simulink library "ForcesSubsystem"  (R2021b)
settings: Solver=VariableStepAuto  StartTime=0.0  StopTime=10.0  RelTol=1e-3
undefined symbols (not defined in the file): sigbuilder_block
libraries: gravitySubsystem x1
settings Model: Creator=mat  LastModifiedBy=mat

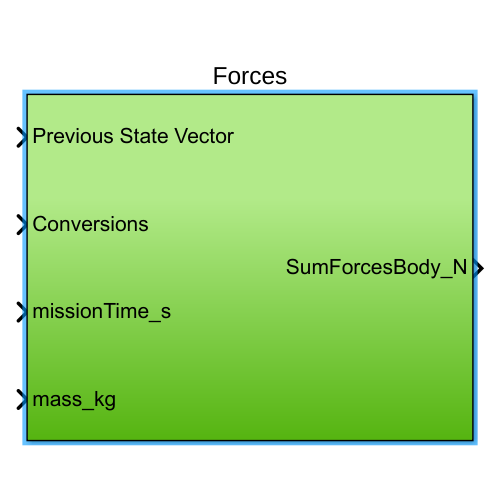
[thumbnail: Simulink's stored preview of the top-level diagram]
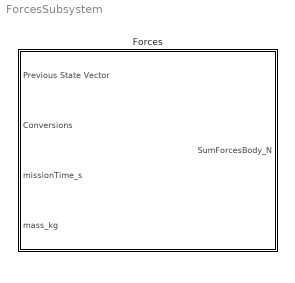
== system ForcesSubsystem ==
  Forces : Subsystem

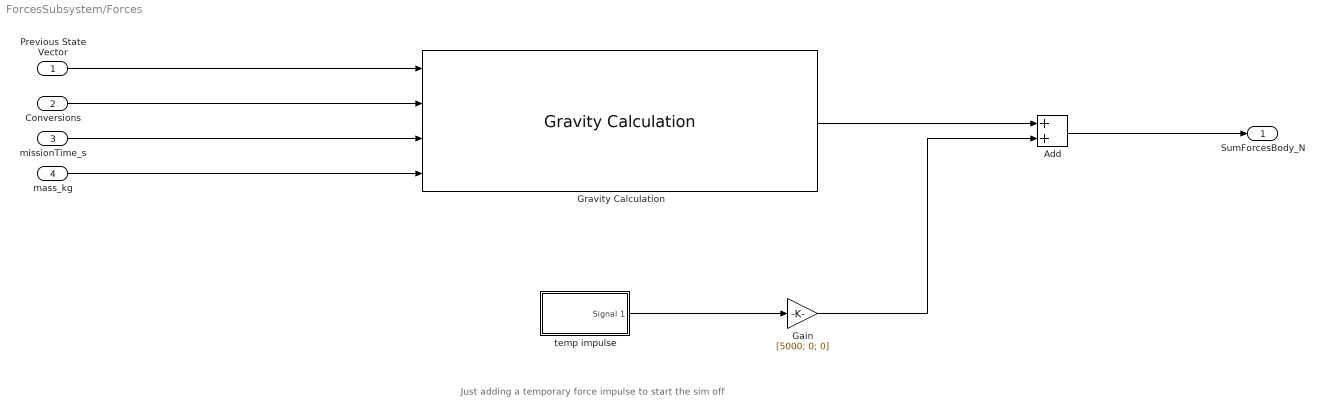
== system ForcesSubsystem/Forces ==
  note: Just adding a temporary force impulse to start the sim off
  Previous State Vector : Inport  OutDataTypeStr=Bus: StateVector_BusType
  Conversions : Inport  Port=2  OutDataTypeStr=Bus: Conversions_BusType
  missionTime_s : Inport  Port=3
  mass_kg : Inport  Port=4
  Add : Sum  InputSameDT=on
  Gain : Gain  Gain=[5000; 0; 0]
  Gravity Calculation : gravitySubsystem/Gravity Calculation  SystemSampleTime=-1  VariantActivationTime=update diagram  Latency=0  AutoFrameSizeCalculation=off
  temp impulse : Subsystem  Tag=STV Subsys  LoadFcn=sigbuilder_block('load');  StartFcn=sigbuilder_block('start');  StopFcn=sigbuilder_block('stop');  ClipboardFcn=sigbuilder_block('clipboard');  mask(Sigbuilder block){tuvar=[0:10]}
      mask help: Simulink:masks:SigbuilderBlock_MD
      mask init:
      | if ~strcmp(get_param(bdroot(gcbh),'SimulationStatus'),'stopped') tuvar = sigbuilder_block('maskInit'); end
      settings: CopyFcn=sigbuilder_block('copy');  DeleteFcn=sigbuilder_block('delete');  ModelCloseFcn=sigbuilder_block('modelClose');  PreSaveFcn=sigbuilder_block('preSave');  PauseFcn=sigbuilder_block('pause');  ContinueFcn=sigbuilder_block('continue');  NameChangeFcn=sigbuilder_block('namechange');  OpenFcn=sigbuilder_block('open',[0 0 1561.26 692.716 ]);  CloseFcn=sigbuilder_block('close');
      mask Display: plot(0, 0, 100, 100,[2, 2, 32, 32, 2], [68, 8, 8, 68, 68],[32, 2], [38, 38], [32, 19, 2],[53, 60, 44], [32, 17, 17, 2],[16, 16, 31, 31]);txt = getActiveGroup(gcbh);text(2, 100, txt,'verticalAlignment', 'top');
  SumForcesBody_N : Outport
  wires:
  mass_kg/1 -> Gravity Calculation/4
  missionTime_s/1 -> Gravity Calculation/3
  Gravity Calculation/1 -> Add/1
  Conversions/1 -> Gravity Calculation/2
  Previous State Vector/1 -> Gravity Calculation/1
  temp impulse/1(Signal 1) -> Gain/1
  Gain/1 -> Add/2
  Add/1 -> SumForcesBody_N/1

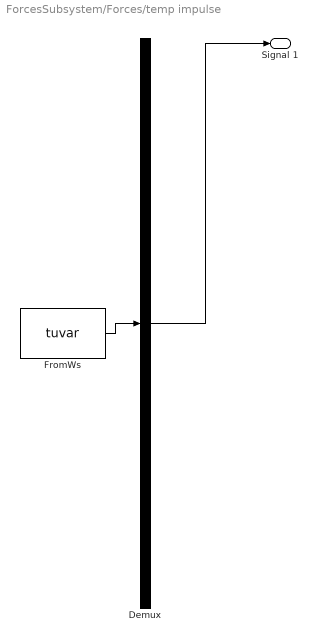
== system ForcesSubsystem/Forces/temp impulse ==
  Demux : Demux  Tag=STV Demux  Outputs=1
      settings: DisplayOption=none
  FromWs : FromWorkspace  Tag=STV FromWs  VariableName=tuvar
      SigBuilderData=|
      | common.afterFinalStr = 'Extrapolate'
      | common.sampleTime = 0
      | dataSet.timeRange = [0 10]
      | dataSet.name = 'Group 1'
      | sbobj.Groups.Name = 'Group 1'
      | sbobj.Groups.Signals.Name = 'Signal 1'
      | sbobj.Groups.Signals.XData = [0 5.01 5.01 10]
      | sbobj.Groups.Signals.YData = [1 1 0 0]
  Signal 1 : Outport  Tag=STV Outport
  wires:
  Demux/1 -> Signal 1/1
  FromWs/1 -> Demux/1
